simulink model "ksrbl_4k4t_hdtrig"  (Simulink 6.2)
settings: Solver=ode45  StartTime=0.0  StopTime=20000  RelTol=1e-3
libraries: xbsIndex_r3 x1214, casper_library x120, xps_library x20
(part 14 of 26)

== system ksrbl_4k4t_hdtrig/pfb_fir_real/pol1_in3_first_tap/pfb_coeff_gen ==
  din : Inport  Port=1  LatchInput=off
  sync : Inport  Port=2  LatchInput=off
  Concat : xbsIndex_r3/Concat  num_inputs=4  explicit_period=off  period=1  dbl_ovrd=off
  Counter : xbsIndex_r3/Counter  cnt_type=Free Running  n_bits=10  bin_pt=0  arith_type=Unsigned  start_count=0  cnt_to=Inf  cnt_by_val=1  operation=Up  explicit_period=on  period=1  load_pin=off  rst=on  en=off  dbl_ovrd=off  show_param=off  use_rpm=on  gen_core=off
      settings: xl_area=[0, 0, 0, 0, 0, 0, 0]
  Delay : xbsIndex_r3/Delay  latency=bram_latency+1  reg_retiming=off  explicit_period=off  period=1  en=off  accept_only_valid=off  init_zero=on  dbl_ovrd=off  show_param=off
      settings: xl_area=[0, 0, 0, 0, 0, 0, 0]
  Delay1 : xbsIndex_r3/Delay  latency=5  reg_retiming=off  explicit_period=off  period=1  en=off  accept_only_valid=off  init_zero=on  dbl_ovrd=off  show_param=off
      settings: xl_area=[0, 0, 0, 0, 0, 0, 0]
  ROM1 : xbsIndex_r3/ROM  depth=1024  initVector=[-1.95360449193984e-005 -5.86373824824353e-005 -9.77787809695406e-005 -0.000136961519242798 -0.000176186878536004 -0.000215456142407859 -0.000254770596694927 -0.000294131529464561 -0.000333540230967701 -0.000372997993591441 -0.000412506111811566 -0.000452065882144957 -0.000491678603101768 -0.000531345575137634 -0.00057106810060559 -0.000610847483707977 -0.000650685030448226 -0.000690582048582418 -0.000730539847570823 -0.000770559738529316 -0.000810643034180581 -0.000850791048805284 -0.000891005098193145 -0.000931286499593767 -0.000971636571667522 -0.00101205663443616 -0.00105254800923341 -0.00109311201865547 -0.00113374998651128 -0.00117446323777281 -0.00121525309852519 -0.00125612089591668 -0.0012970679581086 -0.00133809561422518 -0.00137920519430318 -0.00142039802924154 -0.00146167545075082 -0.00150303879130263 -0.00154448938407893 -0.00158602856292113 -0.00162765766227924 -0.00166937801716091 -0.00171119096308017 -0.00175309783600636 -0.00179509997231278 -0.00183719870872528 -0.00187939538227079 -0.00192169133022575 -0.00196408789006439 -0.00200658639940705 -0.00204918819596824 -0.00209189461750476 -0.00213470700176369 -0.00217762668643021 -0.00222065500907546 -0.00226379330710427 -0.00230704291770274 -0.00235040517778589 -0.00239388142394503 -0.00243747299239523 -0.00248118121892266 -0.00252500743883177 -0.00256895298689248 -0.00261301919728732 -0.00265720740355837 -0.00270151893855428 -0.00274595513437711 -0.00279051732232913 -0.00283520683285961 -0.00288002499551139 -0.00292497313886758 -0.00297005259049806 -0.00301526467690592 -0.0030606107234739 -0.00310609205441077 -0.00315170999269754 -0.0031974658600337 -0.00324336097678347 -0.00328939666192177 -0.00333557423298038 -0.00338189500599389 -0.00342836029544561 -0.00347497141421356 -0.00352172967351617 -0.00356863638285814 -0.00361569284997621 -0.00366290038078473 -0.00371026027932139 -0.0037577738476928 -0.00380544238601998 -0.00385326719238395 -0.00390124956277108 -0.00394939079101858 -0.00399769216875989 -0.00404615498536995 -0.00409478052791051 -0.00414357008107548 -0.00419252492713603 -0.00424164634588582 -0.00429093561458624 -0.00434039400791139 -0.0043900227978933 -0.0044398232538669 -0.00448979664241511 -0.00453994422731382 -0.00459026726947688 -0.00464076702690103 -0.00469144475461088 -0.00474230170460374 -0.00479333912579457 -0.00484455826396084 -0.00489596036168731 -0.00494754665831095 -0.00499931838986565 -0.0050512767890271 -0.00510342308505753 -0.00515575850375045 -0.00520828426737544 -0.00526100159462291 -0.00531391170054876 -0.00536701579651917 -0.00542031509015529 -0.00547381078527795 -0.00552750408185238 -0.00558139617593287 -0.00563548825960751 -0.0056897815209429 -0.00574427714392879 -0.00579897630842278 -0.00585388019009512 -0.00590898996037331 -0.00596430678638681 -0.00601983183091183 -0.006075566252316 -0.00613151120450307 -0.00618766783685775 -0.00624403729419033 -0.00630062071668158 -0.00635741923982739 -0.00641443399438365 -0.00647166610631106 -0.0065291166967199 -0.00658678688181488 -0.00664467777284005 -0.00670279047602365 -0.00676112609252295 -0.00681968571836934 -0.00687847044441308 -0.00693748135626846 -0.00699671953425864 -0.0070561860533608 -0.00711588198315117 -0.00717580838775008 -0.00723596632576712 -0.00729635685024632 -0.00735698100861126 -0.00741783984261036 -0.00747893438826213 -0.00754026567580047 -0.00760183472962001 -0.00766364256822145 -0.00772569020415702 -0.00778797864397599 -0.00785050888817004 -0.00791328193111896 -0.00797629876103618 -0.00803956035991441 -0.00810306770347134 -0.00816682176109544 -0.00823082349579168 -0.00829507386412747 -0.00835957381617844 -0.00842432429547453 -0.00848932623894594 -0.0085545805768692 -0.00862008823281334 -0.00868585012358606 -0.00875186715917999 -0.00881814024271899 -0.00888467027040459 -0.00895145813146234 -0.00901850470808845 -0.00908581087539623 -0.00915337750136286 -0.00922120544677606 -0.00928929556518085 -0.00935764870282646 -0.00942626569861328 -0.00949514738403984 ...(+16644 chars)]  arith_type="Signed  (2's comp)"  n_bits=8  bin_pt=7  latency=4  init_zero=on  explicit_period=off  period=1  rst=off  init_reg=0  en=off  dbl_ovrd=off  show_param=on  distributed_mem=off  use_rpm=on  gen_core=off
      settings: xl_area=[0, 0, 0, 0, 0, 0, 0]
  ROM2 : xbsIndex_r3/ROM  depth=1024  initVector=[0.000263994494270992 0.000793790765333044 0.00132599846643037 0.00186061964024239 0.00239765630500669 0.00293711045444783 0.00347898405770716 0.00402327905927222 0.00456999737890649 0.00511914091157999 0.00567071152739955 0.0062247110715397 0.00678114136417345 0.0073400042004041 0.00790130135019662 0.0084650345583097 0.00903120554422771 0.00959981600209368 0.0101708676006419 0.0107443619831309 0.0113203007672771 0.0118986855451885 0.0124795178832987 0.0130627993223009 0.0136485313770831 0.0142367155366628 0.014827353264122 0.015420445996543 0.0160159951449443 0.0166140020942168 0.0172144682030597 0.0178173948039183 0.0184227832029204 0.0190306346798139 0.0196409504879044 0.0202537318539937 0.0208689799783179 0.0214866960344859 0.0221068811694188 0.022729536503289 0.0233546631294603 0.0239822621144271 0.0246123344977557 0.0252448812920241 0.0258799034827636 0.0265174020283999 0.0271573778601946 0.0277998318821875 0.0284447649711389 0.0290921779764717 0.0297420717202153 0.0303944469969483 0.0310493045737422 0.0317066451901058 0.0323664695579295 0.0330287783614295 0.0336935722570932 0.034360851873625 0.0350306178118914 0.0357028706448674 0.0363776109175828 0.0370548391470693 0.0377345558223073 0.0384167614041735 0.0391014563253891 0.0397886409904673 0.0404783157756628 0.0411704810289198 0.0418651370698219 0.0425622841895416 0.0432619226507901 0.043964052687768 0.0446686745061159 0.0453757882828655 0.0460853941663909 0.0467974922763607 0.04751208270369 0.0482291655104935 0.0489487407300372 0.0496708083666933 0.0503953683958929 0.0511224207640799 0.0518519653886663 0.0525840021579864 0.0533185309312521 0.0540555515385082 0.0547950637805891 0.0555370674290745 0.0562815622262462 0.0570285478850452 0.0577780240890295 0.0585299904923315 0.0592844467196164 0.0600413923660409 0.0608008269972125 0.0615627501491482 0.0623271613282347 0.0630940600111889 0.0638634456450179 0.0646353176469804 0.0654096754045475 0.0661865182753654 0.0669658455872166 0.067747656637983 0.0685319506956086 0.069318726998063 0.0701079847533053 0.0708997231392475 0.07169394130372 0.072490638364436 0.0732898134089569 0.0740914654946582 0.0748955936486955 0.0757021968679712 0.0765112741191012 0.0773228243383828 0.078136846431762 0.0789533392748019 0.079772301712651 0.0805937325600128 0.0814176306011148 0.0822439945896786 0.0830728232488894 0.0839041152713679 0.0847378693191406 0.085574084023611 0.0864127579855325 0.0872538897749797 0.0880974779313221 0.0889435209631962 0.0897920173484802 0.0906429655342672 0.0914963639368401 0.0923522109416458 0.0932105049032716 0.0940712441454197 0.0949344269608841 0.0958000516115267 0.0966681163282548 0.0975386193109979 0.0984115587286858 0.0992869327192269 0.100164739389487 0.101044976815268 0.101927643041288 0.10281273608116 0.103700253917375 0.10459019450128 0.10548255575306 0.106377335561721 0.107274531785071 0.108174142249702 0.109076164750975 0.109980597053002 0.110887436888629 0.111796681959423 0.112708329935654 0.113622378456283 0.114538825128943 0.115457667529932 0.116378903204193 0.117302529665305 0.118228544395467 0.119156944845491 0.120087728434784 0.121020892551342 0.121956434551735 0.122894351761102 0.123834641473134 0.124777300950071 0.125722327422687 0.126669718090289 0.127619470120701 0.12857158065026 0.12952604678381 0.130482865594692 0.131442034124742 0.132403549384278 0.133367408352103 0.134333607975495 0.135302145170201 0.136273016820437 0.137246219778883 0.13822175086668 0.139199606873424 0.140179784557169 0.141162280644421 0.142147091830138 0.143134214777731 0.144123646119059 0.145115382454434 0.146109420352617 0.147105756350824 0.148104386954722 0.149105308638433 0.150108517844537 0.151114010984075 0.15212178443655 0.153131834549932 0.154144157640663 0.155158749993659 0.156175607862319 0.157194727468525 0.158216105002653 0.159239736623576 0.160265618458675 0.161293746603839 0.16232411712348 0.163356726050539 0.164391569386493 0.165428643101365 0.166467943133735 0.167509465390747 0.168553205748125 ...(+14479 chars)]  arith_type="Signed  (2's comp)"  n_bits=8  bin_pt=7  latency=4  init_zero=on  explicit_period=off  period=1  rst=off  init_reg=0  en=off  dbl_ovrd=off  show_param=on  distributed_mem=off  use_rpm=on  gen_core=off
      settings: xl_area=[0, 0, 0, 0, 0, 0, 0]
  ROM3 : xbsIndex_r3/ROM  depth=1024  initVector=[0.999999396380429 0.999995041050674 0.999986465752932 0.999973670570085 0.999956655625658 0.999935421083817 0.99990996714937 0.999880294067759 0.99984640212506 0.999808291647981 0.999765963003855 0.999719416600634 0.999668652886887 0.999613672351793 0.999554475525133 0.999491062977285 0.999423435319215 0.999351593202471 0.999275537319172 0.999195268402001 0.999110787224194 0.99902209459953 0.998929191382323 0.998832078467406 0.998730756790122 0.998625227326313 0.998515491092304 0.998401549144894 0.998283402581337 0.998161052539332 0.998034500197004 0.997903746772894 0.997768793525938 0.997629641755452 0.997486292801116 0.997338748042957 0.997187008901328 0.997031076836892 0.996870953350601 0.996706639983679 0.996538138317598 0.996365449974063 0.996188576614982 0.996007519942454 0.995822281698739 0.995632863666241 0.995439267667479 0.995241495565069 0.995039549261695 0.994833430700085 0.994623141862989 0.994408684773147 0.994190061493268 0.993967274126 0.993740324813905 0.993509215739426 0.993273949124865 0.993034527232348 0.992790952363801 0.992543226860913 0.992291353105111 0.992035333517529 0.99177517055897 0.991510866729883 0.991242424570321 0.990969846659914 0.990693135617834 0.990412294102759 0.990127324812841 0.989838230485666 0.989545013898223 0.989247677866866 0.988946225247277 0.988640658934428 0.988330981862544 0.988017197005064 0.987699307374604 0.987377316022914 0.987051226040841 0.986721040558288 0.986386762744172 0.986048395806385 0.98570594299175 0.985359407585976 0.985008792913622 0.984654102338047 0.98429533926137 0.983932507124424 0.98356560940671 0.983194649626353 0.982819631340057 0.982440558143055 0.982057433669066 0.981670261590245 0.981279045617136 0.980883789498623 0.980484497021881 0.980081172012329 0.979673818333574 0.979262439887368 0.978847040613551 0.978427624490003 0.978004195532591 0.977576757795118 0.977145315369266 0.976709872384547 0.976270433008247 0.975827001445372 0.975379581938593 0.97492817876819 0.974472796251999 0.974013438745352 0.973550110641021 0.973082816369163 0.97261156039726 0.972136347230062 0.971657181409525 0.971174067514757 0.970687010161955 0.970196014004345 0.969701083732123 0.96920222407239 0.968699439789097 0.968192735682974 0.967682116591477 0.967167587388718 0.966649152985403 0.96612681832877 0.965600588402525 0.965070468226772 0.964536462857953 0.96399857738878 0.963456816948169 0.962911186701173 0.962361691848915 0.961808337628519 0.961251129313045 0.960690072211416 0.960125171668353 0.959556433064302 0.958983861815368 0.958407463373241 0.957827243225125 0.95724320689367 0.956655359936896 0.956063707948126 0.955468256555906 0.954869011423939 0.954265978251006 0.953659162770897 0.953048570752331 0.952434207998884 0.951816080348916 0.951194193675488 0.950568553886293 0.949939166923577 0.949306038764059 0.948669175418857 0.948028582933408 0.947384267387391 0.946736234894645 0.946084491603094 0.945429043694665 0.944769897385204 0.944107058924405 0.943440534595719 0.942770330716277 0.942096453636809 0.941418909741559 0.940737705448203 0.940052847207769 0.939364341504547 0.938672194856012 0.937976413812733 0.937277004958294 0.936573974909204 0.935867330314814 0.935157077857231 0.934443224251229 0.933725776244164 0.933004740615887 0.932280124178656 0.931551933777046 0.930820176287862 0.930084858620051 0.92934598771461 0.928603570544498 0.927857614114547 0.927108125461368 0.926355111653263 0.925598579790131 0.92483853700338 0.924074990455831 0.923307947341628 0.922537414886144 0.921763400345887 0.920985911008407 0.920204954192203 0.919420537246628 0.918632667551791 0.917841352518467 0.917046599587998 0.916248416232196 0.915446809953251 0.91464178828363 0.913833358785982 0.913021529053039 0.91220630670752 0.911387699402031 0.910565714818968 0.909740360670417 0.908911644698054 0.908079574673046 0.907244158395953 0.906405403696623 0.905563318434095 0.904717910496498 0.903869187800945 0.903017158293436 0.902161829948755 0.901303210770364 0.900441308790305 0.899576132069092 ...(+14488 chars)]  arith_type="Signed  (2's comp)"  n_bits=8  bin_pt=7  latency=4  init_zero=on  explicit_period=off  period=1  rst=off  init_reg=0  en=off  dbl_ovrd=off  show_param=off  distributed_mem=off  use_rpm=on  gen_core=off
      settings: xl_area=[0, 0, 0, 0, 0, 0, 0]
  ROM4 : xbsIndex_r3/ROM  depth=1024  initVector=[-0.00026330631403908 -0.000788114004277693 -0.00131051687776899 -0.00183051707608281 -0.00234811676486496 -0.00286331813376437 -0.00337612339636068 -0.0038865347900909 -0.00439455457617581 -0.00490018503954674 -0.00540342848877141 -0.00590428725597985 -0.00640276369678972 -0.00689886019023205 -0.00739257913867597 -0.00788392296775371 -0.00837289412628479 -0.0088594950862008 -0.00934372834246916 -0.00982559641301676 -0.0103051018386539 -0.0107822471829973 -0.0112570350323932 -0.0117294679958402 -0.0121995487049117 -0.0126672798136784 -0.0131326639986305 -0.013595703958599 -0.0140564024146778 -0.0145147621101451 -0.0149707858103839 -0.015424476302804 -0.0158758363967615 -0.0163248689234802 -0.0167715767359711 -0.0172159627089529 -0.0176580297387715 -0.0180977807433197 -0.0185352186619564 -0.0189703464554258 -0.0194031671057763 -0.019833683616279 -0.0202618990113463 -0.0206878163364502 -0.0211114386580405 -0.0215327690634618 -0.0219518106608722 -0.02236856657916 -0.0227830399678613 -0.0231952339970764 -0.0236051518573875 -0.0240127967597745 -0.0244181719355317 -0.0248212806361841 -0.0252221261334032 -0.025620711718923 -0.0260170407044553 -0.0264111164216055 -0.0268029422217878 -0.0271925214761398 -0.0275798575754378 -0.0279649539300114 -0.0283478139696579 -0.0287284411435566 -0.0291068389201829 -0.0294830107872225 -0.0298569602514849 -0.030228690838817 -0.0305982060940166 -0.0309655095807459 -0.0313306048814439 -0.0316934955972402 -0.032054185347867 -0.0324126777715721 -0.0327689765250309 -0.0331230852832595 -0.0334750077395256 -0.0338247476052614 -0.0341723086099749 -0.0345176945011618 -0.0348609090442166 -0.0352019560223442 -0.0355408392364709 -0.0358775625051555 -0.0362121296645005 -0.0365445445680617 -0.0368748110867602 -0.0372029331087919 -0.037528914539538 -0.0378527593014753 -0.0381744713340858 -0.0384940545937674 -0.0388115130537425 -0.0391268507039686 -0.0394400715510472 -0.0397511796181335 -0.0400601789448451 -0.0403670735871718 -0.0406718676173837 -0.0409745651239411 -0.0412751702114022 -0.0415736870003322 -0.0418701196272118 -0.0421644722443454 -0.0424567490197695 -0.0427469541371606 -0.0430350917957434 -0.0433211662101989 -0.0436051816105716 -0.0438871422421778 -0.044167052365513 -0.0444449162561593 -0.0447207382046927 -0.0449945225165907 -0.0452662735121391 -0.0455359955263395 -0.0458036929088161 -0.0460693700237223 -0.0463330312496481 -0.0465946809795262 -0.0468543236205393 -0.0471119635940259 -0.0473676053353875 -0.0476212532939942 -0.0478729119330917 -0.0481225857297071 -0.0483702791745552 -0.0486159967719442 -0.0488597430396824 -0.0491015225089833 -0.049341339724372 -0.0495791992435906 -0.0498151056375042 -0.0500490634900064 -0.0502810773979246 -0.050511151970926 -0.0507392918314226 -0.0509655016144767 -0.0511897859677063 -0.0514121495511906 -0.0516325970373744 -0.0518511331109739 -0.052067762468882 -0.0522824898200726 -0.052495319885506 -0.0527062573980341 -0.0529153071023048 -0.0531224737546672 -0.0533277621230761 -0.0535311769869973 -0.0537327231373119 -0.0539324053762208 -0.0541302285171502 -0.0543261973846553 -0.0545203168143254 -0.0547125916526884 -0.0549030267571152 -0.0550916269957245 -0.0552783972472868 -0.0554633424011292 -0.05564646735704 -0.0558277770251726 -0.0560072763259502 -0.0561849701899703 -0.0563608635579088 -0.0565349613804244 -0.056707268618063 -0.056877790241162 -0.0570465312297548 -0.0572134965734745 -0.0573786912714589 -0.0575421203322544 -0.0577037887737205 -0.0578637016229337 -0.0580218639160923 -0.0581782806984203 -0.0583329570240718 -0.0584858979560355 -0.0586371085660387 -0.0587865939344516 -0.058934359150192 -0.0590804093106292 -0.0592247495214887 -0.0593673848967562 -0.0595083205585823 -0.0596475616371866 -0.0597851132707625 -0.0599209806053811 -0.0600551687948962 -0.0601876830008484 -0.0603185283923699 -0.0604477101460885 -0.060575233446033 -0.060701103483537 -0.060825325457144 -0.0609479045725117 -0.0610688460423172 -0.0611881550861612 -0.0613058369304731 -0.0614218968084157 ...(+16613 chars)]  arith_type="Signed  (2's comp)"  n_bits=8  bin_pt=7  latency=4  init_zero=on  explicit_period=off  period=1  rst=off  init_reg=0  en=off  dbl_ovrd=off  show_param=off  distributed_mem=off  use_rpm=on  gen_core=off
      settings: xl_area=[0, 0, 0, 0, 0, 0, 0]
  Register : xbsIndex_r3/Register  init=0  reg_only_valid=off  explicit_period=off  period=1  rst=off  en=off  out_en=off  dbl_ovrd=off  show_param=off
      settings: xl_area=[0, 0, 0, 0, 0, 0, 0]
  Reinterpret{1..4} (4 alike) : xbsIndex_r3/Reinterpret  force_arith_type=on  arith_type=Unsigned  force_bin_pt=on  bin_pt=0  force_valid=on
  dout : Outport
  sync_out : Outport  Port=2
  coeff : Outport  Port=3
  wires:
  din/1 -> Delay1/1
  Delay1/1 -> dout/1
  sync/1 -> Counter/1, Delay/1
  Delay/1 -> sync_out/1
  Concat/1 -> Register/1
  Register/1 -> coeff/1
  Counter/1 -> ROM1/1, ROM2/1, ROM3/1, ROM4/1
  ROM1/1 -> Reinterpret1/1
  Reinterpret1/1 -> Concat/1
  ROM2/1 -> Reinterpret2/1
  Reinterpret2/1 -> Concat/2
  ROM3/1 -> Reinterpret3/1
  Reinterpret3/1 -> Concat/3
  ROM4/1 -> Reinterpret4/1
  Reinterpret4/1 -> Concat/4
